simulink model "RocketSE"  (R2017b)
settings: Solver=FixedStepAuto  StartTime=0.0  StopTime=30  FixedStep=Tau  RelTol=1e-3
values from neighbouring files (symbols this model uses):
  Ad = expm(A*T)    [KalmanBSP.m]    (also in ReadARISData.m = expm(A*Tau); SEFromData.m = expm(A*Tau); SEFromDataWithGPS.m = expm(A*Tau); SEFromDataWithPressure.m = expm(A*Tau))
  B = [0;0;0]    [KalmanBSP.m]    (also in ReadARISData.m = [0;0;0;0;0]; SEFromData.m = [0;0;0;0;0;0]; SEFromDataWithGPS.m; SEFromDataWithPressure.m = [0;0;0;0;0;0])
  C = [1 0 0;0 0 1]    [KalmanBSP.m]    (also in ReadARISData.m = [1 0 0 0 0; 0 0 1 -1 0;0 0 0 0 1]; SEFromData.m = [1 0 0 0 0 0;0 0 1 0 0 0;0 0 0 1 0 0;0 0 0 1 0 0;0 0 0 0 1 0; SEFromDataWithGPS.m; SEFromDataWithPressure.m = [0 0 1 0 0 0;0 0 0 1 0 0;0 0 0 1 0 0;0 0 0 0 1 0])
  D = [0;0]    [KalmanBSP.m]    (also in ReadARISData.m = [0]; SEFromData.m; SEFromDataWithGPS.m; SEFromDataWithPressure.m)
  R = 8.314    [CalcPressure.m]    (also in KalmanBSP.m = [varp 0;0 vara]; ReadARISData.m = diag([2^32;MACL;2^32]); SEFromData.m = [1 0 0 0 0;0 12 0 0 0;0 0 15 0 0;0 0 0 1 0;0 0 0 0 1]; SEFromDataWithGPS.m = diag([GPSvar ACLvar]))
  Time = 0:0.001:30    [KalmanBSP.m]
undefined symbols (not defined in the file or in its folder): Discrete
libraries: ctrlSharedLib x1
settings Model: Creator=geilomat  LastModifiedBy=geilomat

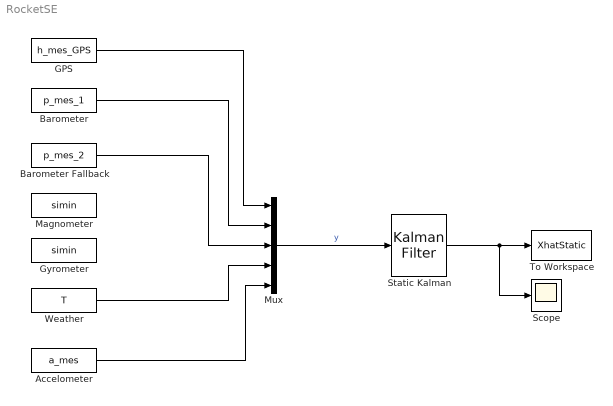
== system RocketSE ==
  Accelometer : FromWorkspace  VariableName=a_mes  SampleTime=0
  "Barometer " : FromWorkspace  VariableName=p_mes_1  SampleTime=0
  "Barometer Fallback " : FromWorkspace  VariableName=p_mes_2  SampleTime=0
  "GPS " : FromWorkspace  VariableName=h_mes_GPS  SampleTime=0.0005  Interpolate=off  OutputAfterFinalValue=Holding final value
  "Gyrometer " : FromWorkspace  VariableName=simin  SampleTime=0
  "Magnometer " : FromWorkspace  VariableName=simin  SampleTime=0
  Mux : Mux  Inputs=5
  Scope : Scope
  Static Kalman : ctrlSharedLib/Kalman Filter  TimeDomain=Discrete-Time  UseCurrentEstimator=on  ModelSource=Individual A, B, C, D matrices  ModelSourceVariable=ss(0.95,1,1,0,1)  A=Ad  B=B  C=C  D=D  NumberOfStates=1  NumberOfInputs=1  NumberOfOutputs=1  InitialEstimateSource=Dialog  X0=0  P0=10  UseK=off  UseGH=off  NumberOfProcessNoiseInputs=1  G=1  TimeInvariantG=on  H=0  TimeInvariantH=on  Q=Q  TimeInvariantQ=on  R=R  TimeInvariantR=on  N=0  TimeInvariantN=on  AddInputPort=off  AddEnablePort=off  OutputEstimatedY=off  OutputP=off  Ts=-1
      settings: SourceProductBaseCode=CT
  To Workspace : ToWorkspace  VariableName=XhatStatic  SaveFormat=Structure With Time  SampleTime=-1
  "Weather " : FromWorkspace  VariableName=T  SampleTime=0
  wires:
  Mux/1 -> Static Kalman/1  "y"
  Accelometer/1 -> Mux/5
  "GPS "/1 -> Mux/1
  "Barometer "/1 -> Mux/2
  "Barometer Fallback "/1 -> Mux/3
  "Weather "/1 -> Mux/4
  Static Kalman/1 -> To Workspace/1, Scope/1
